simulink model "sim1"  (R2016b)
settings: Solver=FixedStepAuto  StartTime=0.0  StopTime=50  FixedStep=0.0001  RelTol=1e-3
settings Model: Creator=lenovo  LastModifiedBy=lenovo

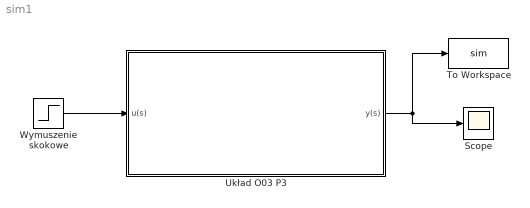
== system sim1 ==
  Scope : Scope
  To Workspace : ToWorkspace  VariableName=sim  SaveFormat=Timeseries  SampleTime=-1
  Układ O03 P3 : Subsystem
      mask Display:
      | color('red')
      | %opis parametrów
      | text(0.3,0.75,'Gx(s) [T=2, k=1]')
      | text(0.3,0.50,'Gy(s) [T=1, k=4]')
      | text(0.3,0.25,'Gz(s) [T=3, k=2]')
      | %opis wejść/wyjść
      | port_label('output', 1, 'y(t)')
      | port_label('input', 1, 'u(t)')
  Wymuszenie skokowe : Step  SampleTime=0
  wires:
  Wymuszenie skokowe/1 -> Układ O03 P3/1(u(s))
  Układ O03 P3/1(y(s)) -> To Workspace/1, Scope/1

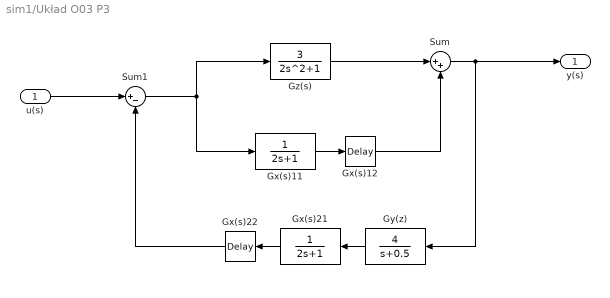
== system sim1/Układ O03 P3 ==
  u(s) : Inport
  Gx(s)11 : TransferFcn  Denominator=[2 1]
  Gx(s)12 : TransportDelay  DelayTime=0.8
  Gx(s)21 : TransferFcn  Denominator=[2 1]
  Gx(s)22 : TransportDelay  DelayTime=0.8
  Gy(z) : TransferFcn  Numerator=[4]  Denominator=[1 0.5]
  Gz(s) : TransferFcn  Numerator=[3]  Denominator=[2 0 1]
  Sum : Sum  Inputs=|++
  Sum1 : Sum  Inputs=|+-
  y(s) : Outport
  wires:
  Sum1/1 -> Gx(s)11/1, Gz(s)/1
  u(s)/1 -> Sum1/1
  Gz(s)/1 -> Sum/1
  Gx(s)12/1 -> Sum/2
  Gx(s)11/1 -> Gx(s)12/1
  Sum/1 -> y(s)/1, Gy(z)/1
  Gx(s)21/1 -> Gx(s)22/1
  Gx(s)22/1 -> Sum1/2
  Gy(z)/1 -> Gx(s)21/1
